simulink model "Fig513"  (R2014b)
settings: Solver=ode3  StartTime=0.0  StopTime=.128  FixedStep=1e-3  RelTol=1e-3
libraries: commseqgen2 x2, simulink_extras x1
settings Model: Creator=Silage  LastModifiedBy=Silage

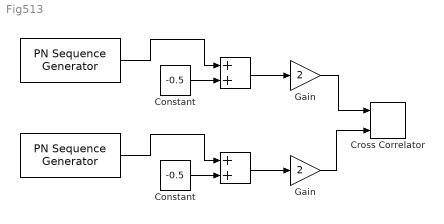
== system Fig513 ==
  " " : commseqgen2/PN Sequence Generator  poly=[1 0 0 1 1]  ini_sta=[1 0 0 1]  outBitMaskSource=Dialog parameter  shift=0  outVarSiz=off  maxOutSizeMode=Dialog parameter  maxOutSize=[10 1]  Ts=1e-3  frameBased=off  sampPerFrame=1  reset=off  bitPackedOutputs=off  outDataType=double  numPackedBits=8  bitPackDataSigned=off  bitPackedOutDType=double
  "    " : Sum
  "     " : commseqgen2/PN Sequence Generator  poly=[1 1 0 0 1]  ini_sta=[1 0 0 1]  outBitMaskSource=Dialog parameter  shift=0  outVarSiz=off  maxOutSizeMode=Dialog parameter  maxOutSize=[10 1]  Ts=1e-3  frameBased=off  sampPerFrame=1  reset=off  bitPackedOutputs=off  outDataType=double  numPackedBits=8  bitPackDataSigned=off  bitPackedOutDType=double
  "       " : Sum
  " Constant " : Constant  Value=-0.5
  " Gain " : Gain  Gain=2
  Constant : Constant  Value=-0.5
  Cross Correlator : simulink_extras/Additional Sinks/Cross Correlator  npts=128  HowOften=128  sampleT=1e-3
  Gain : Gain  Gain=2
  wires:
  " "/1 -> "    "/1
  Constant/1 -> "    "/2
  "    "/1 -> Gain/1
  Gain/1 -> Cross Correlator/1
  "     "/1 -> "       "/1
  " Constant "/1 -> "       "/2
  "       "/1 -> " Gain "/1
  " Gain "/1 -> Cross Correlator/2
